simulink library "Clutch"  (R2017a)
settings: Solver=VariableStepAuto  StartTime=0.0  StopTime=10.0  RelTol=1e-3
undefined symbols (not defined in the file): clt, Clutch, Engine, lib_Clutch_Final
libraries: autolibutils x4, autolibdrivetraincommon x3, autolibcoupling x2, simulink x1, lib_Clutch_2017a x1, lib_Clutch x1
settings Model: Creator=leste  LastModifiedBy=Vraj M

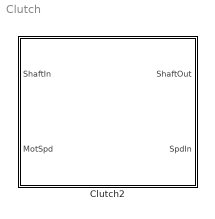
== system Clutch ==
  Clutch2 : Subsystem  AncestorBlock=lib_Clutch_Final/Clutch
      mask Display:
      | image('Images/Clutch.jpg')
      | color('red');
      | port_label('Input',1,'ShaftIn');
      | port_label('Input',2,'SpdOut');
      | port_label('Output',1,'ShaftOut');
      | port_label('Output',2,'SpdIn');

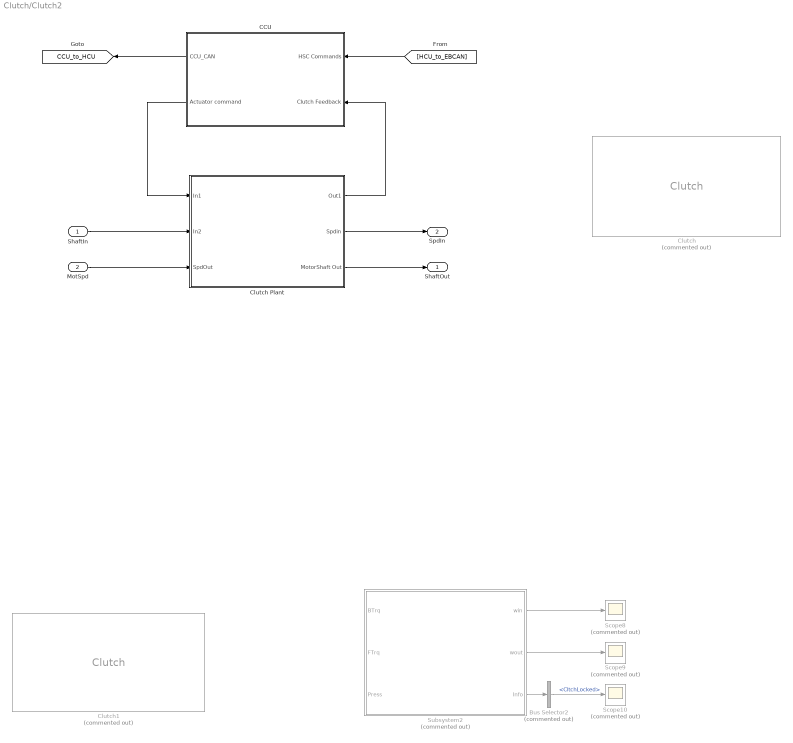
== system Clutch/Clutch2 ==
  ShaftIn : Inport
  MotSpd : Inport  Port=2
  Bus Selector2 : BusSelector  Commented=on  OutputSignals=Cltch.CltchLocked
  CCU : Subsystem
      mask Display: image('SoftECU.jpg')
  Clutch : lib_Clutch_2017a/Clutch  Commented=on  SystemSampleTime=-1
  Clutch Plant : Subsystem
      mask Display:
      | image('Images/Clutch.jpg')
      | color('red');
      | port_label('Input',2,'ShaftIn');
      | port_label('Input',3,'SpdOut');
      | port_label('Output',3,'ShaftOut');
      | port_label('Output',2,'SpdIn');
  Clutch1 : lib_Clutch/Clutch  Commented=on  SystemSampleTime=-1
  Scope10 : Scope  Commented=on
  Scope8 : Scope  Commented=on
  Scope9 : Scope  Commented=on
  Subsystem2 : Subsystem  Commented=on  mask{Reff=0.121, Ndisk=1, Aeff=0.02129, Jin=Engine.Inertia + (0.75*clt.plant.init.inertia), Jout=.1 + (0.25*clt.plant.init.inertia), muk=0.25, mus=0.3, bin=.001*2, bout=.001*2, win_o=0, wout_o=0, tauC=0.01*10, maxAbsSpd=3000, InitiallyLocked=on}
      mask prompts: Reff "Clutch force radius"; Ndisk "Number of disks"; Aeff "Pressure area"; Jin "Input Shaft inertia"; Jout "output Shaft inertia"; muk "Kinetic FC"; mus "Static FC"; bin "Input shaft damping"; bout "Output shaft damping"; win_o "Initial input shaft velocity"; wout_o "Initial output shaft velocity"; tauC "Clutch actuation time constant"; maxAbsSpd "max output speed"; InitiallyLocked "Clutch initially locked"
  ShaftOut : Outport
  SpdIn : Outport  Port=2
  tag scope: CCU_to_HCU=global
  wires:
  Subsystem2/1(win) -> Scope8/1
  Subsystem2/2(wout) -> Scope9/1
  Subsystem2/3(Info) -> Bus Selector2/1
  Bus Selector2/1 -> Scope10/1  "<CltchLocked>"
  [HCU_to_EBCAN] -> CCU/1(HSC Commands)
  CCU/2("Actuator command ") -> Clutch Plant/1(In1)
  ShaftIn/1 -> Clutch Plant/2(In2)
  MotSpd/1 -> Clutch Plant/3(SpdOut)
  Clutch Plant/2(Spdin) -> SpdIn/1
  Clutch Plant/3(MotorShaft Out) -> ShaftOut/1
  CCU/1("CCU_CAN ") -> [CCU_to_HCU]
  Clutch Plant/1(Out1) -> CCU/2(Clutch Feedback)

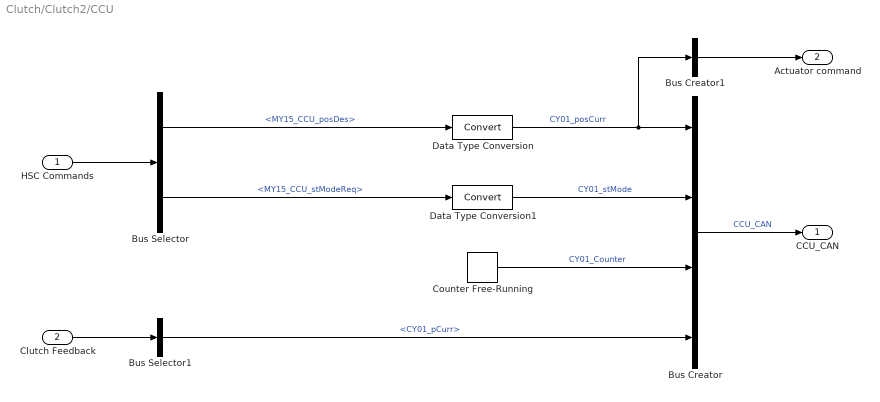
== system Clutch/Clutch2/CCU ==
  HSC Commands : Inport
  Clutch Feedback : Inport  Port=2
  Bus Creator : BusCreator  Inputs=4
  Bus Creator1 : BusCreator  Inputs=1
  Bus Selector : BusSelector  OutputSignals=MY15_CCU_posDes,MY15_CCU_stModeReq
  Bus Selector1 : BusSelector  OutputSignals=CY01_pCurr
  Counter Free-Running : simulink/Sources/Counter Free-Running  NumBits=15  tsamp=-1
  Data Type Conversion : DataTypeConversion
  Data Type Conversion1 : DataTypeConversion
  "CCU_CAN " : Outport
  "Actuator command " : Outport  Port=2
  wires:
  Bus Selector1/1 -> Bus Creator/4  "<CY01_pCurr>"
  HSC Commands/1 -> Bus Selector/1
  Bus Selector/1 -> Data Type Conversion/1  "<MY15_CCU_posDes>"
  Data Type Conversion/1 -> Bus Creator1/1, Bus Creator/1  "CY01_posCurr"
  Bus Creator/1 -> "CCU_CAN "/1  "CCU_CAN"
  Bus Creator1/1 -> "Actuator command "/1
  Counter Free-Running/1 -> Bus Creator/3  "CY01_Counter"
  Bus Selector/2 -> Data Type Conversion1/1  "<MY15_CCU_stModeReq>"
  Data Type Conversion1/1 -> Bus Creator/2  "CY01_stMode"
  Clutch Feedback/1 -> Bus Selector1/1

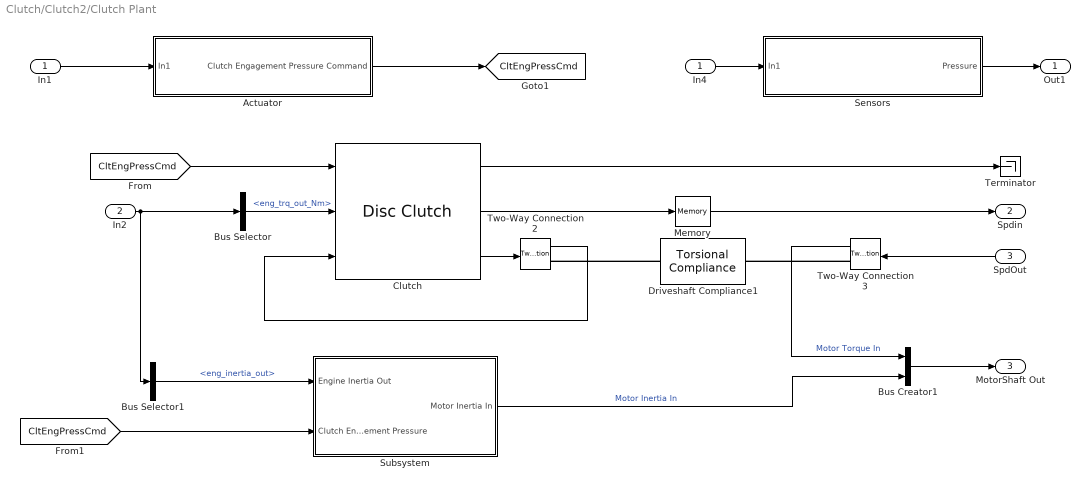
== system Clutch/Clutch2/Clutch Plant ==
  In1 : Inport
  In2 : Inport  Port=2
  SpdOut : Inport  Port=3
  " Actuator" : Subsystem
  " Sensors " : Subsystem
  Bus Creator1 : BusCreator  Inputs=2
  Bus Selector : BusSelector  OutputSignals=eng_trq_out_Nm
  Bus Selector1 : BusSelector  OutputSignals=eng_inertia_out
  Clutch : autolibcoupling/Disc Clutch  port_config=Simulink  Reff=0.121  Ndisk=1  Aeff=0.02129  Jin=Engine.Inertia + (0.75*clt.plant.init.inertia)  Jout=.1 + (0.25*clt.plant.init.inertia)  muk=0.25  mus=0.3  bin=.001*2  bout=.001*2  win_o=0  wout_o=0  tauC=0.01*10  InitiallyLocked=on  maxAbsSpd=3000  blkID=1
      settings: SourceProductName=Powertrain Blockset  SourceProductBaseCode=PW
  Driveshaft Compliance1 : autolibcoupling/Torsional Compliance  port_config=Two-way connection  k=1000000  b=100  theta_o=0  domega_o=0  omega_c=100  blkID=0
      settings: SourceProductName=Powertrain Blockset
  In4 : InportShadow
  Memory : Memory
  Subsystem : Subsystem
  Terminator : Terminator
  Two-Way Connection2 : TwoWayConnection
  Two-Way Connection3 : TwoWayConnection
  Out1 : Outport
  Spdin : Outport  Port=2
  MotorShaft Out : Outport  Port=3
  tag scope: CltEngPressCmd=global
  wires:
  Subsystem/1(Motor Inertia In) -> Bus Creator1/2  "Motor Inertia In"
  Bus Creator1/1 -> MotorShaft Out/1
  Bus Selector1/1 -> Subsystem/1(Engine Inertia Out)  "<eng_inertia_out>"
  [CltEngPressCmd] -> Subsystem/2(Clutch Engagement Pressure)
  Clutch/2 -> Memory/1
  Two-Way Connection3/1 -> Bus Creator1/1  "Motor Torque In"
  Two-Way Connection2/1 -> Clutch/3
  Memory/1 -> Spdin/1
  In2/1 -> Bus Selector/1, Bus Selector1/1
  SpdOut/1 -> Two-Way Connection3/1
  Clutch/3 -> Two-Way Connection2/1
  In1/1 -> " Actuator"/1(In1)
  Clutch/1 -> Terminator/1
  " Actuator"/1(Clutch Engagement Pressure Command) -> [CltEngPressCmd]
  [CltEngPressCmd] -> Clutch/1
  Bus Selector/1 -> Clutch/2  "<eng_trq_out_Nm>"
  In4/1 -> " Sensors "/1(In1)
  " Sensors "/1(Pressure) -> Out1/1
  connections:
  Two-Way Connection3/RConn1 -- Driveshaft Compliance1/RConn1
  Driveshaft Compliance1/LConn1 -- Two-Way Connection2/RConn1

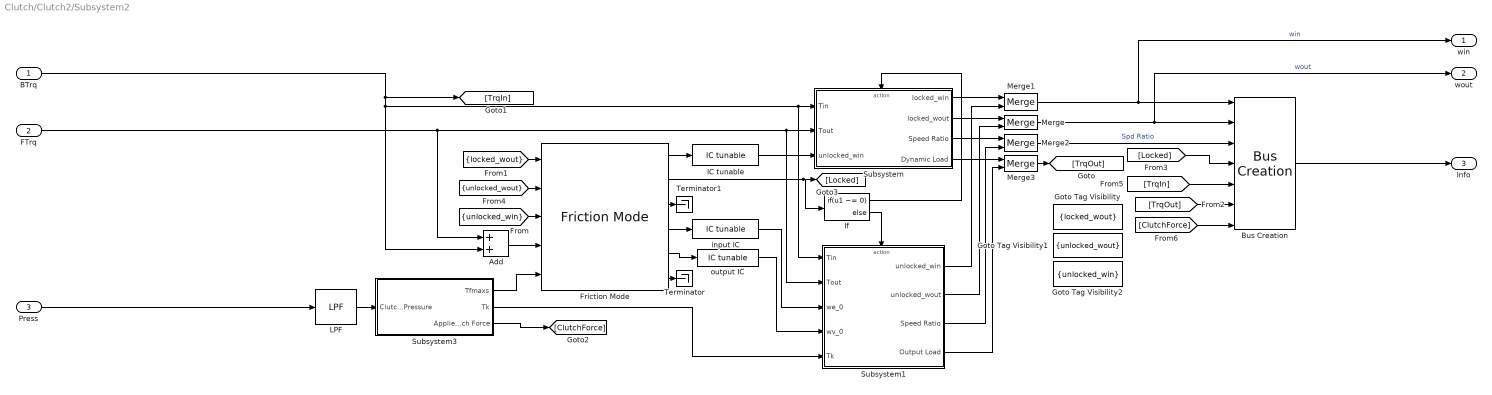
== system Clutch/Clutch2/Subsystem2 ==
  BTrq : Inport
  FTrq : Inport  Port=2
  Press : Inport  Port=3
  Add : Sum
  Bus Creation : autolibdrivetraincommon/Dry Clutch/Bus Creation
      settings: SourceProductName=Powertrain Blockset  SourceProductBaseCode=PW
  Friction Mode : autolibdrivetraincommon/Dry Clutch/Friction Mode
      settings: SourceProductName=Powertrain Blockset  SourceProductBaseCode=PW
  Goto Tag Visibility : GotoTagVisibility  GotoTag=locked_wout
  Goto Tag Visibility1 : GotoTagVisibility  GotoTag=unlocked_wout
  Goto Tag Visibility2 : GotoTagVisibility  GotoTag=unlocked_win
  IC tunable : autolibutils/IC tunable  IC=win_o
      settings: SourceProductName=Powertrain Blockset  SourceProductBaseCode=PW
  If : If  IfExpression=u1 ~= 0
  LPF : autolibdrivetraincommon/Dry Clutch/LPF  OverrideUsingVariant=1
      settings: SourceProductName=Powertrain Blockset  SourceProductBaseCode=PW
  Merge{,1..3} (4 alike) : Merge
  Subsystem : Subsystem
  Subsystem1 : Subsystem
  Subsystem3 : Subsystem
  Terminator : Terminator
  Terminator1 : Terminator
  input IC : autolibutils/IC tunable  IC=win_o
      settings: SourceProductName=Powertrain Blockset  SourceProductBaseCode=PW
  output IC : autolibutils/IC tunable  IC=wout_o
      settings: SourceProductName=Powertrain Blockset  SourceProductBaseCode=PW
  win : Outport
  wout : Outport  Port=2
  Info : Outport  Port=3
  wires:
  [Locked] -> Bus Creation/4
  FTrq/1 -> Subsystem1/2(Tout), Subsystem/2(Tout), Add/1
  [unlocked_win] -> Friction Mode/3
  Bus Creation/1 -> Info/1
  [TrqOut] -> Bus Creation/6
  Friction Mode/2 -> [Locked], If/1
  Subsystem/1(locked_win) -> Merge1/1
  Subsystem1/1(unlocked_win) -> Merge1/2
  Merge3/1 -> [TrqOut]
  [locked_wout] -> Friction Mode/1
  [unlocked_wout] -> Friction Mode/2
  Subsystem/4(Dynamic Load) -> Merge3/1
  Subsystem1/4(Output Load) -> Merge3/2
  Friction Mode/1 -> IC tunable/1
  IC tunable/1 -> Subsystem/3(unlocked_win)
  Merge2/1 -> Bus Creation/3  "Spd Ratio"
  input IC/1 -> Subsystem1/3(we_0)
  Subsystem1/2(unlocked_wout) -> Merge/2
  output IC/1 -> Subsystem1/4(wv_0)
  If/2 -> Subsystem1/Action
  LPF/1 -> Subsystem3/1(Clutch Pressure)
  Merge1/1 -> win/1, Bus Creation/1  "win"
  Friction Mode/4 -> input IC/1
  Friction Mode/5 -> output IC/1
  Subsystem/3(Speed Ratio) -> Merge2/1
  Subsystem3/3(Applied Clutch Force) -> [ClutchForce]
  Merge/1 -> wout/1, Bus Creation/2  "wout"
  Subsystem1/3(Speed Ratio) -> Merge2/2
  Press/1 -> LPF/1
  Subsystem/2(locked_wout) -> Merge/1
  If/1 -> Subsystem/Action
  BTrq/1 -> [TrqIn], Subsystem1/1(Tin), Subsystem/1(Tin), Add/2
  Friction Mode/3 -> Terminator1/1
  Add/1 -> Friction Mode/4
  [ClutchForce] -> Bus Creation/7
  Friction Mode/6 -> Terminator/1
  Subsystem3/2(Tk) -> Subsystem1/5(Tk)
  [TrqIn] -> Bus Creation/5
  Subsystem3/1(Tfmaxs) -> Friction Mode/5

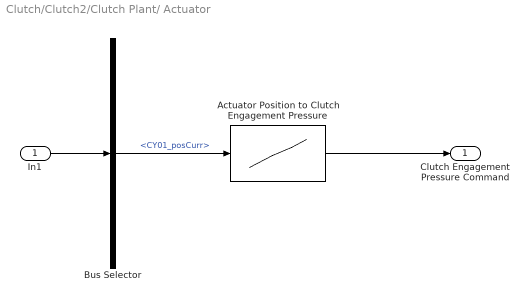
== system Clutch/Clutch2/Clutch Plant/ Actuator ==
  In1 : Inport
  Actuator Position to Clutch Engagement Pressure : Lookup_n-D  NumberOfTableDimensions=1  BreakpointsForDimension1=|  Table=|  InternalRulePriority=Speed  RndMeth=Simplest  InputSameDT=on
      BreakpointsForDimension1=|
      | [0
      | 100
      | 200
      | 300
      | 400
      | 500
      | 600
      | 700
      | 800
      | 900
      | 1000
      | 1100
      | 1200
      | 1300
      | 1400
      | 1500
      | 1600
      | 1700
      | 1800
      | 1900
      | 2000
      | 2100
      | 2200
      | 2300
      | 2400
      | 2500
      | 2600
      | 2700
      | 2800
      | 2900
      | 3000
      | 3100
      | 3200
      | 3300
      | 3400
      | 3500
      | 3600
      | 3700
      | 3800
      | 3900
      | 4000
      | 4100
      | 4200
      | 4300
      | 4400
      | 4500
      | 4600
      | 4700
      | 4800
      | 4900
      | 5000
      | 5100
      | 5200
      | 5300
      | 5400
      | 5500
      | 5600
      | 5700
      | 5800
      | 5900
      | 6000
      | 6100
      | 6200
      | 6300
      | 6400
      | 
      | ]
      Table=|
      | [892800
      | 892800
      | 892800
      | 833280
      | 773760
      | 714240
      | 654720
      | 595200
      | 535680
      | 476160
      | 416640
      | 357120
      | 297600
      | 238080
      | 178560
      | 119040
      | 59520
      | 0
      | 0
      | 0
      | 0
      | 0
      | 0
      | 0
      | 0
      | 0
      | 0
      | 0
      | 0
      | 0
      | 0
      | 0
      | 0
      | 0
      | 0
      | 0
      | 0
      | 0
      | 0
      | 0
      | 0
      | 0
      | 0
      | 0
      | 0
      | 0
      | 0
      | 0
      | 0
      | 0
      | 0
      | 0
      | 0
      | 0
      | 0
      | 0
      | 0
      | 0
      | 0
      | 0
      | 0
      | 0
      | 0
      | 0
      | 0
      | 
      | 
      | ]
  Bus Selector : BusSelector  OutputSignals=CY01_posCurr
  Clutch Engagement Pressure Command : Outport
  wires:
  In1/1 -> Bus Selector/1
  Bus Selector/1 -> Actuator Position to Clutch Engagement Pressure/1  "<CY01_posCurr>"
  Actuator Position to Clutch Engagement Pressure/1 -> Clutch Engagement Pressure Command/1

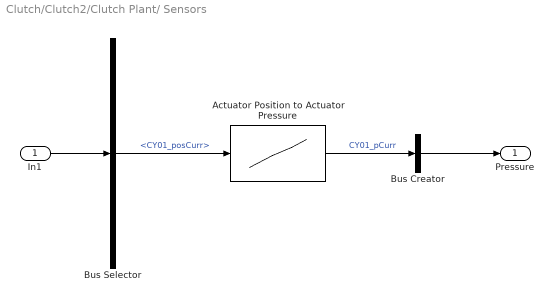
== system Clutch/Clutch2/Clutch Plant/ Sensors  ==
  In1 : Inport
  Actuator Position to Actuator Pressure : Lookup_n-D  NumberOfTableDimensions=1  BreakpointsForDimension1=|  Table=|  InternalRulePriority=Speed  RndMeth=Simplest  InputSameDT=on
      BreakpointsForDimension1=|
      | [0
      | 300
      | 400
      | 500
      | 600
      | 700
      | 800
      | 900
      | 1000
      | 1100
      | 1200
      | 1300
      | 1400
      | 1500
      | 1600
      | 1700
      | 1800
      | 1900
      | 2000
      | 2100
      | 2200
      | 2300
      | 2400
      | 2500
      | 2600
      | 2700
      | 2800
      | 2900
      | 3000
      | 3100
      | 3200
      | 3300
      | 3400
      | 3500
      | 3600
      | 3700
      | 3800
      | 3900
      | 4000
      | 4100
      | 4200
      | 4300
      | 4400
      | 4500
      | 4600
      | 4650
      | ]
      Table=|
      | [0.4
      | 1.2
      | 2.6
      | 4
      | 5.6
      | 6.8
      | 8.6
      | 10.4
      | 12.2
      | 14
      | 15.8
      | 17.4
      | 18.8
      | 19.6
      | 20.2
      | 20
      | 19.8
      | 19.6
      | 19
      | 18.8
      | 18.4
      | 18
      | 17.8
      | 17.6
      | 17.4
      | 17.2
      | 17
      | 16.8
      | 16.6
      | 16.6
      | 16.6
      | 16.8
      | 17
      | 17.2
      | 17.4
      | 17.8
      | 18
      | 18.4
      | 18.6
      | 19
      | 19.4
      | 20.4
      | 21.2
      | 25.4
      | 36.4
      | 41
      | ]
  Bus Creator : BusCreator  Inputs=1
  Bus Selector : BusSelector  OutputSignals=CY01_posCurr
  Pressure : Outport
  wires:
  Actuator Position to Actuator Pressure/1 -> Bus Creator/1  "CY01_pCurr"
  Bus Selector/1 -> Actuator Position to Actuator Pressure/1  "<CY01_posCurr>"
  In1/1 -> Bus Selector/1
  Bus Creator/1 -> Pressure/1

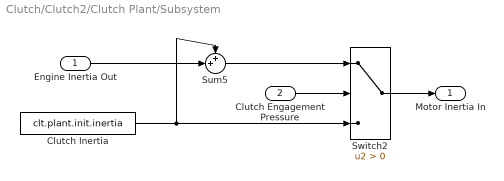
== system Clutch/Clutch2/Clutch Plant/Subsystem ==
  Engine Inertia Out : Inport
  Clutch Engagement Pressure : Inport  Port=2
  Clutch Inertia : Constant  Value=clt.plant.init.inertia
  Sum5 : Sum  Inputs=++|  SaturateOnIntegerOverflow=on  InputSameDT=on  OutDataTypeStr=Inherit: Same as first input
  Switch2 : Switch  Criteria=u2 > Threshold  SaturateOnIntegerOverflow=on  InputSameDT=on
  Motor Inertia In : Outport
  wires:
  Clutch Engagement Pressure/1 -> Switch2/2
  Clutch Inertia/1 -> Sum5/1, Switch2/3
  Sum5/1 -> Switch2/1
  Engine Inertia Out/1 -> Sum5/2
  Switch2/1 -> Motor Inertia In/1

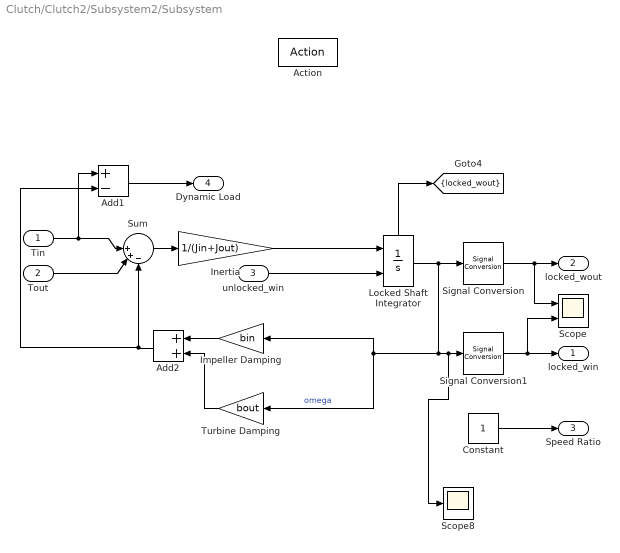
== system Clutch/Clutch2/Subsystem2/Subsystem ==
  Tin : Inport
  Tout : Inport  Port=2
  unlocked_win : Inport  Port=3
  Action : ActionPort  InitializeStates=reset
  Add1 : Sum  Inputs=+-
  Add2 : Sum
  Constant : Constant
  Impeller Damping : Gain  Gain=bin  SaturateOnIntegerOverflow=on  OutDataTypeStr=Inherit: Same as input  ParamDataTypeStr=Inherit: Same as input
  Inertia : Gain  Gain=1/(Jin+Jout)  SaturateOnIntegerOverflow=on  OutDataTypeStr=Inherit: Same as input  ParamDataTypeStr=Inherit: Same as input
  Locked Shaft Integrator : Integrator  InitialConditionSource=external  LimitOutput=on  UpperSaturationLimit=maxAbsSpd  LowerSaturationLimit=-maxAbsSpd  ShowStatePort=on  ZeroCross=off
  Scope : Scope  NumInputPorts=2
  Scope8 : Scope
  Signal Conversion : SignalConversion  OverrideOpt=off
  Signal Conversion1 : SignalConversion  OverrideOpt=off
  Sum : Sum  Inputs=||++-  SaturateOnIntegerOverflow=on  InputSameDT=on  OutDataTypeStr=Inherit: Same as first input
  Turbine Damping : Gain  Gain=bout  SaturateOnIntegerOverflow=on  OutDataTypeStr=Inherit: Same as input  ParamDataTypeStr=Inherit: Same as input
  locked_win : Outport  InitialOutput=win_o
  locked_wout : Outport  Port=2  InitialOutput=win_o
  Speed Ratio : Outport  Port=3  InitialOutput=1
  Dynamic Load : Outport  Port=4  InitialOutput=0
  tag scope: locked_wout=scoped
  wires:
  Tin/1 -> Sum/1, Add1/1
  Inertia/1 -> Locked Shaft Integrator/1
  Sum/1 -> Inertia/1
  Locked Shaft Integrator/1 -> Signal Conversion/1, Signal Conversion1/1, Scope8/1, Impeller Damping/1, Turbine Damping/1  "omega"
  Tout/1 -> Sum/2
  Constant/1 -> Speed Ratio/1
  Signal Conversion1/1 -> Scope/2, locked_win/1
  unlocked_win/1 -> Locked Shaft Integrator/2
  Impeller Damping/1 -> Add2/1
  Add2/1 -> Sum/3, Add1/2
  Locked Shaft Integrator/State -> [locked_wout]
  Turbine Damping/1 -> Add2/2
  Add1/1 -> Dynamic Load/1
  Signal Conversion/1 -> Scope/1, locked_wout/1

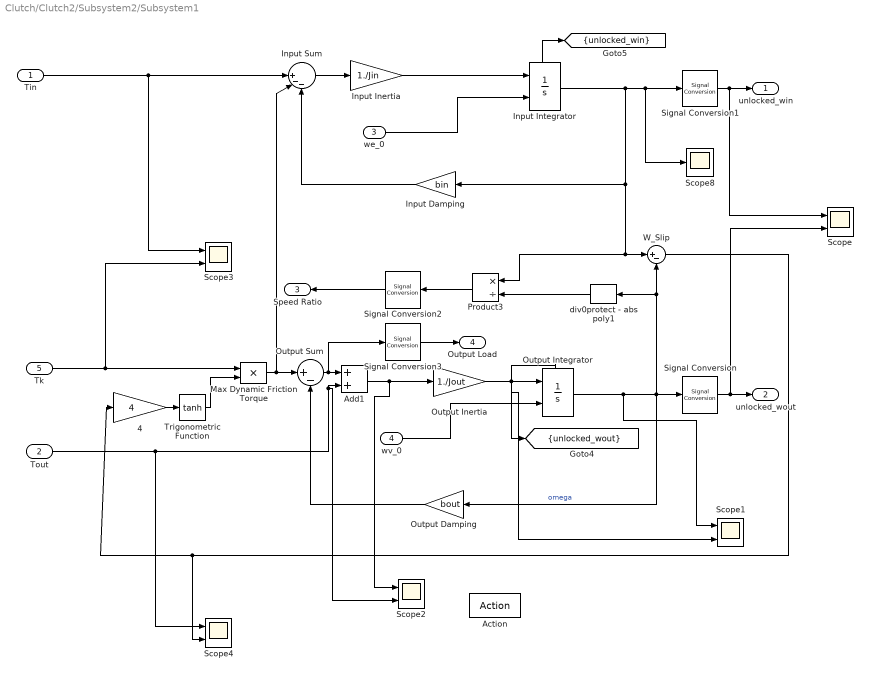
== system Clutch/Clutch2/Subsystem2/Subsystem1 ==
  Tin : Inport
  Tout : Inport  Port=2
  we_0 : Inport  Port=3
  wv_0 : Inport  Port=4
  Tk : Inport  Port=5
  Action : ActionPort  InitializeStates=reset
  4 : Gain  Gain=4  SaturateOnIntegerOverflow=on  OutDataTypeStr=Inherit: Same as input  ParamDataTypeStr=Inherit: Same as input
  Add1 : Sum
  Input Damping : Gain  Gain=bin  SaturateOnIntegerOverflow=on  OutDataTypeStr=Inherit: Same as input  ParamDataTypeStr=Inherit: Same as input
  Input Inertia : Gain  Gain=1./Jin  SaturateOnIntegerOverflow=on  OutDataTypeStr=Inherit: Same as input  ParamDataTypeStr=Inherit: Same as input
  Input Integrator : Integrator  InitialConditionSource=external  LimitOutput=on  UpperSaturationLimit=maxAbsSpd  LowerSaturationLimit=-maxAbsSpd  ShowStatePort=on
  Input Sum : Sum  Inputs=||+--  SaturateOnIntegerOverflow=on  InputSameDT=on  OutDataTypeStr=Inherit: Same as first input
  Max Dynamic Friction Torque : Product  SaturateOnIntegerOverflow=on  RndMeth=Zero  InputSameDT=on  OutDataTypeStr=Inherit: Same as first input
  Output Damping : Gain  Gain=bout  SaturateOnIntegerOverflow=on  OutDataTypeStr=Inherit: Same as input  ParamDataTypeStr=Inherit: Same as input
  Output Integrator : Integrator  InitialConditionSource=external  LimitOutput=on  UpperSaturationLimit=maxAbsSpd  LowerSaturationLimit=-maxAbsSpd  ShowStatePort=on
  Output Inertia : Gain  Gain=1./Jout  SaturateOnIntegerOverflow=on  OutDataTypeStr=Inherit: Same as input  ParamDataTypeStr=Inherit: Same as input
  Output Sum : Sum  Inputs=|+-  SaturateOnIntegerOverflow=on  InputSameDT=on  OutDataTypeStr=Inherit: Same as first input
  Product3 : Product  Inputs=*/
  Scope{,1..4} (5 alike) : Scope  NumInputPorts=2
  Scope8 : Scope
  Signal Conversion{,1..3} (4 alike) : SignalConversion  OverrideOpt=off
  Trigonometric Function : Trigonometry  Operator=tanh
  W_Slip : Sum  Inputs=|+-  SaturateOnIntegerOverflow=on  InputSameDT=on  OutDataTypeStr=Inherit: Same as first input
  div0protect - abs poly1 : autolibutils/div0protect - abs poly  thresh=1e-6
      settings: SourceProductName=Powertrain Blockset  SourceProductBaseCode=PW
  unlocked_win : Outport  InitialOutput=win_o
  unlocked_wout : Outport  Port=2  InitialOutput=wout_o
  Speed Ratio : Outport  Port=3  InitialOutput=0
  Output Load : Outport  Port=4  InitialOutput=0
  tag scope: unlocked_win=scoped, unlocked_wout=scoped
  wires:
  Input Integrator/1 -> W_Slip/1, Product3/1, Input Damping/1, Signal Conversion1/1, Scope8/1
  Input Damping/1 -> Input Sum/3
  Input Inertia/1 -> Input Integrator/1
  Signal Conversion3/1 -> Output Load/1
  Output Integrator/1 -> Scope1/1, Signal Conversion/1, Output Damping/1, div0protect - abs poly1/1, W_Slip/2  "omega"
  div0protect - abs poly1/1 -> Product3/2
  Input Integrator/State -> [unlocked_win]
  Trigonometric Function/1 -> Max Dynamic Friction Torque/2
  Tout/1 -> Scope4/1, Scope2/2, Add1/2
  we_0/1 -> Input Integrator/2
  Signal Conversion/1 -> Scope/2, unlocked_wout/1
  Add1/1 -> Scope2/1, Output Inertia/1
  Tin/1 -> Scope3/1, Input Sum/1
  Product3/1 -> Signal Conversion2/1
  Max Dynamic Friction Torque/1 -> Input Sum/2, Output Sum/1
  Input Sum/1 -> Input Inertia/1
  Output Inertia/1 -> Scope1/2, Output Integrator/1
  Output Damping/1 -> Output Sum/2
  Signal Conversion2/1 -> Speed Ratio/1
  Output Sum/1 -> Signal Conversion3/1, Add1/1
  Output Integrator/State -> [unlocked_wout]
  wv_0/1 -> Output Integrator/2
  4/1 -> Trigonometric Function/1
  Tk/1 -> Scope3/2, Max Dynamic Friction Torque/1
  Signal Conversion1/1 -> Scope/1, unlocked_win/1
  W_Slip/1 -> Scope4/2, 4/1

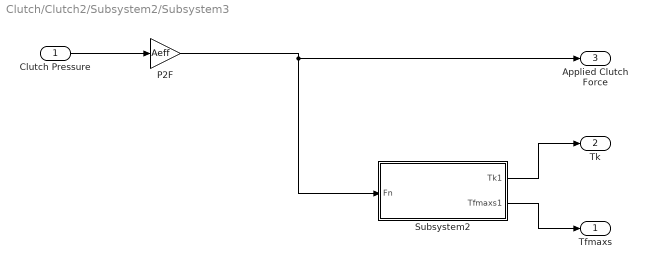
== system Clutch/Clutch2/Subsystem2/Subsystem3 ==
  Clutch Pressure : Inport
  P2F : Gain  Gain=Aeff
  Subsystem2 : Subsystem
  Tfmaxs : Outport
  Tk : Outport  Port=2
  Applied Clutch Force : Outport  Port=3
  wires:
  Subsystem2/1(Tk1) -> Tk/1
  Clutch Pressure/1 -> P2F/1
  Subsystem2/2(Tfmaxs1) -> Tfmaxs/1
  P2F/1 -> Applied Clutch Force/1, Subsystem2/1(Fn)

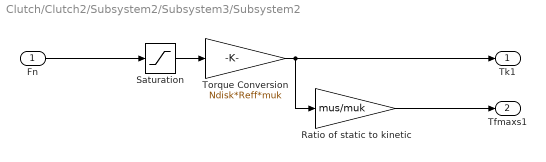
== system Clutch/Clutch2/Subsystem2/Subsystem3/Subsystem2 ==
  Fn : Inport
  Ratio of static to kinetic : Gain  Gain=mus/muk  SaturateOnIntegerOverflow=on  OutDataTypeStr=Inherit: Same as input  ParamDataTypeStr=Inherit: Same as input
  Saturation : Saturate  UpperLimit=inf  LowerLimit=eps
  Torque Conversion : Gain  Gain=Ndisk*Reff*muk  SaturateOnIntegerOverflow=on  OutDataTypeStr=Inherit: Same as input  ParamDataTypeStr=Inherit: Same as input
  Tk1 : Outport  InitialOutput=0
  Tfmaxs1 : Outport  Port=2  InitialOutput=0
  wires:
  Saturation/1 -> Torque Conversion/1
  Fn/1 -> Saturation/1
  Torque Conversion/1 -> Tk1/1, Ratio of static to kinetic/1
  Ratio of static to kinetic/1 -> Tfmaxs1/1
